simulink model "Supervisor_1"  (R2025b)
settings: configuration reference "MCConfiguration" (kept outside this file)
undefined symbols (not defined in the file or in its folder): Targets
settings Model: DataDictionary=embeddedBoard_common.sldd  Creator=rpumpo  LastModifiedBy=rpumpo
settings ConfigSetRef: SourceName=MCConfiguration

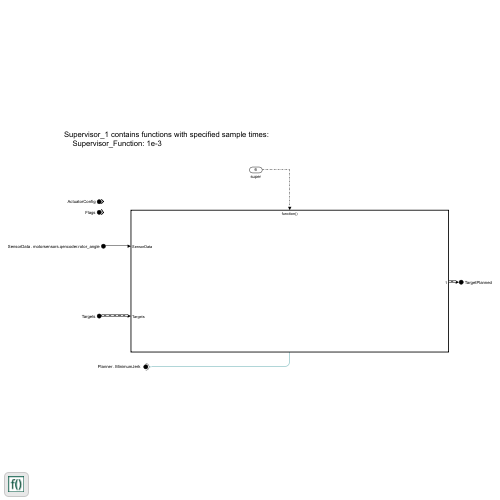
[thumbnail: Simulink's stored preview of the top-level diagram]
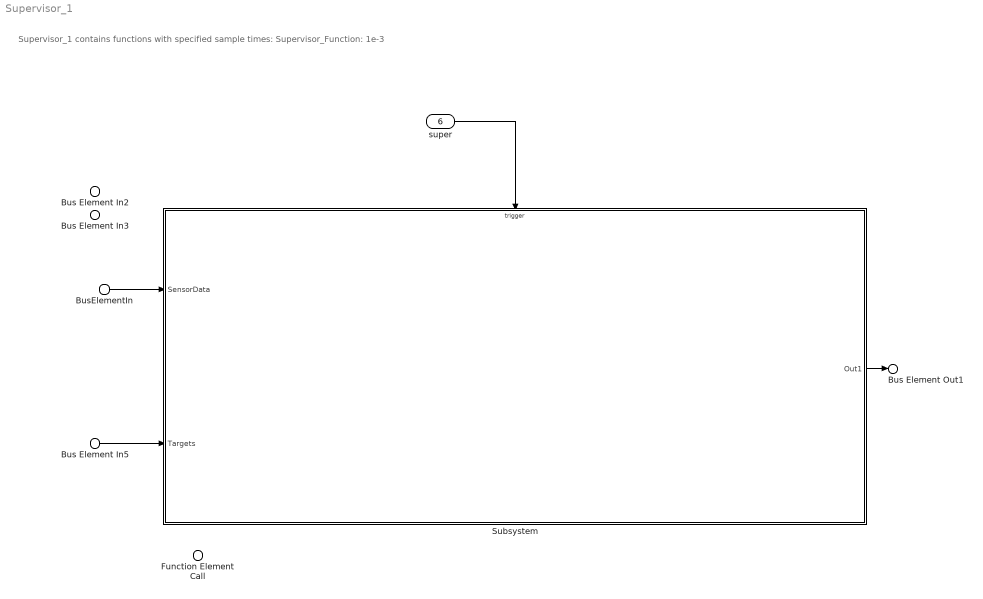
== system Supervisor_1 ==
  note: Supervisor_1 contains functions with specified sample times:
      |  	Supervisor_Function: 1e-3
  Bus Element In2 : Inport  PortName=ActuatorConfig
  Bus Element In3 : Inport  Port=2  PortName=Flags
  BusElementIn : Inport  Description=Mechanical Angle before gearbox  Port=3  PortName=SensorData  Element=motorsensors.qencoder.rotor_angle
  Bus Element In5 : Inport  Port=4  PortName=Targets
  Function Element Call : Inport  Port=5  AllowServiceAccess=on  PortName=Planner  Element=MinimumJerk
  super : Inport  Port=6  SampleTime=1e-3  OutputFunctionCall=on
  Subsystem : Subsystem
  Bus Element Out1 : Outport  PortName=TargetPlanned
  wires:
  Subsystem/1(Out1) -> Bus Element Out1/1
  Bus Element In5/1 -> Subsystem/2(Targets)
  BusElementIn/1 -> Subsystem/1(SensorData)
  super/1 -> Subsystem/Trigger

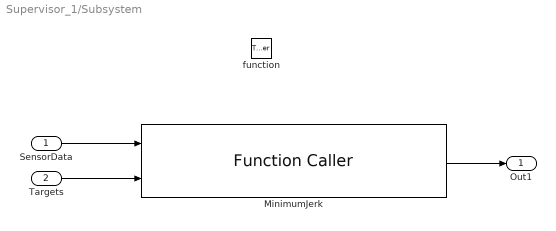
== system Supervisor_1/Subsystem ==
  SensorData : Inport
  Targets : Inport  Port=2
  function : TriggerPort  TriggerType=function-call  VariantControl=(inherit)
  MinimumJerk : FunctionCaller  FunctionPrototype=PlannedTargets = Planner.MinimumJerk(Sensors,Targets)  InputArgumentSpecifications=single(1),Targets  OutputArgumentSpecifications=Targets
  Out1 : Outport
  wires:
  SensorData/1 -> MinimumJerk/1
  Targets/1 -> MinimumJerk/2
  MinimumJerk/1 -> Out1/1
